simulink model "T71"  (R2023b)
settings: Solver=VariableStepAuto  StartTime=0.0  StopTime=10  RelTol=1e-3
settings Model: Creator=Lilian  LastModifiedBy=Lilian

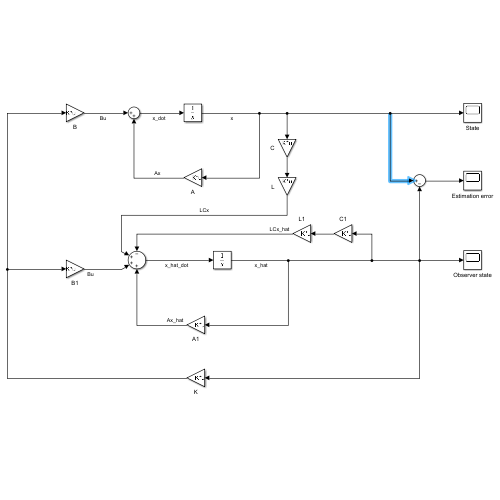
[thumbnail: Simulink's stored preview of the top-level diagram]
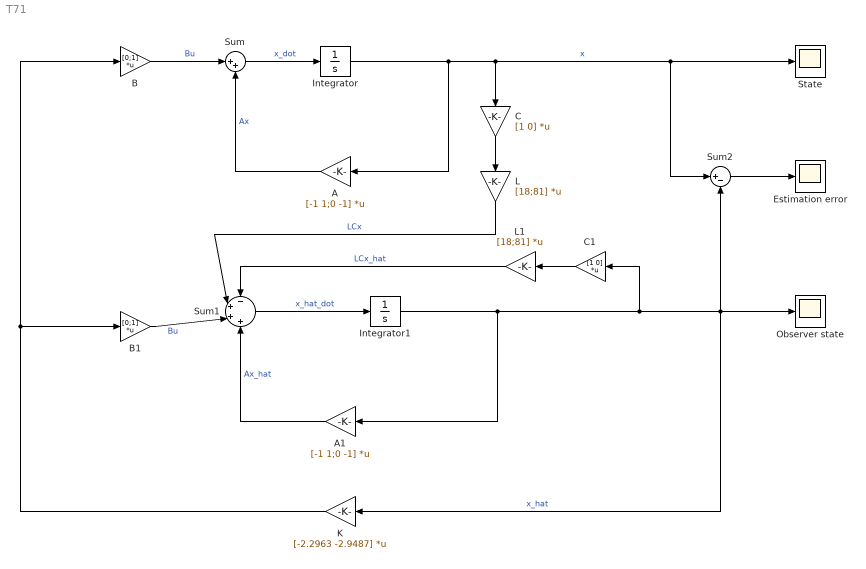
== system T71 ==
  A : Gain  Gain=[-1 1;0 -1]  Multiplication=Matrix(K*u)
  A1 : Gain  Gain=[-1 1;0 -1]  Multiplication=Matrix(K*u)
  B : Gain  Gain=[0;1]  Multiplication=Matrix(K*u)
  B1 : Gain  Gain=[0;1]  Multiplication=Matrix(K*u)
  C : Gain  Gain=[1 0]  Multiplication=Matrix(K*u)
  C1 : Gain  Gain=[1 0]  Multiplication=Matrix(K*u)
  Estimation error : Scope
  Integrator : Integrator  InitialCondition=[1;-1]
  Integrator1 : Integrator  InitialCondition=[0;1]
  K : Gain  Gain=[-2.2963 -2.9487]  Multiplication=Matrix(K*u)
  L : Gain  Gain=[18;81]  Multiplication=Matrix(K*u)
  L1 : Gain  Gain=[18;81]  Multiplication=Matrix(K*u)
  Observer state : Scope
  State : Scope
  Sum : Sum  Inputs=|++
  Sum1 : Sum  Inputs=-+++
  Sum2 : Sum  Inputs=|+-
  wires:
  B/1 -> Sum/1  "Bu"
  Sum/1 -> Integrator/1  "x_dot"
  Integrator/1 -> A/1, C/1, State/1, Sum2/1  "x"
  A/1 -> Sum/2  "Ax"
  Sum1/1 -> Integrator1/1  "x_hat_dot"
  Integrator1/1 -> A1/1, C1/1, K/1, Sum2/2, Observer state/1  "x_hat"
  C/1 -> L/1
  A1/1 -> Sum1/4  "Ax_hat"
  B1/1 -> Sum1/3  "Bu"
  L/1 -> Sum1/2  "LCx"
  C1/1 -> L1/1
  L1/1 -> Sum1/1  "LCx_hat"
  Sum2/1 -> Estimation error/1
  K/1 -> B/1, B1/1
